simulink model "MoordynSimulinkCoupling_Activefloat"  (R2018b)
settings: Solver=ode45  StartTime=0.0  StopTime=100  RelTol=1e-3
InitFcn:
  | cd 'D:\data\40_mahfouz\Moordyn\MoorDyn v1.01.01'
StartFcn:
  | loadlibrary('MoorDyn','MoorDyn')
StopFcn:
  | calllib('MoorDyn','LinesClose'); % close MoorDyn
  | unloadlibrary MoorDyn; % unload library (never forget to do this!)
CloseFcn:
  | calllib('MoorDyn','LinesClose'); % close MoorDyn
  | unloadlibrary MoorDyn; % unload library (never forget to do this!)
settings Model: Creator=mahfouz  LastModifiedBy=mahfouz
settings DataIOCC: SaveOutput=off  SignalLogging=off  DSMLogging=off  VisualizeSimOutput=off  SaveTime=off
settings OptimizationCC: BlockReduction=off  BooleanDataType=off  ConditionallyExecuteInputs=off  OptimizeBlockIOStorage=off  BufferReuse=off  GlobalBufferReuse=off  ExpressionFolding=off  EnableMemcpy=off  LocalBlockOutputs=off  InitFltsAndDblsToZero=on  EfficientMapNaN2IntZero=off  LifeSpan=inf  OptimizeDataStoreBuffers=off  BusAssignmentInplaceUpdate=off
settings DebuggingCC: SFExecutionAtInitializationDiag=none
settings HardwareCC: TargetBitPerPointer=64  TargetBitPerSizeT=64  TargetBitPerPtrDiffT=64  TargetLongLongMode=on  TargetIntDivRoundTo=Zero  TargetEndianess=LittleEndian  TargetWordSize=64  TargetHWDeviceType=MATLAB Host  ProdEqTarget=off
settings RTWCC: SystemTargetFile=matsim.tlc  PackageName=moordyn  TemplateMakefile=matsim_tmf  Description=Simpack MatSIM Target
settings CodeAppCC: StateflowObjectComments=on
settings STFCustomTargetCC: ModelReferenceCompliant=off  MATLABClassNameForMDSCustomization=Simulink.SoftwareTarget.TargetSpecificTriggerConfigurationBase  GRTInterface=on  SystemTargetFile=matsim.tlc
settings ConfigComp: CovHTMLOptions=-sRT=1 -sVT=0 -aTS=1 -bRG=1 -bTC=1 -hTR=0 -nFC=0 -nFD=1 -scm=1 -bcm=1 -xEv=0 -xEM=0

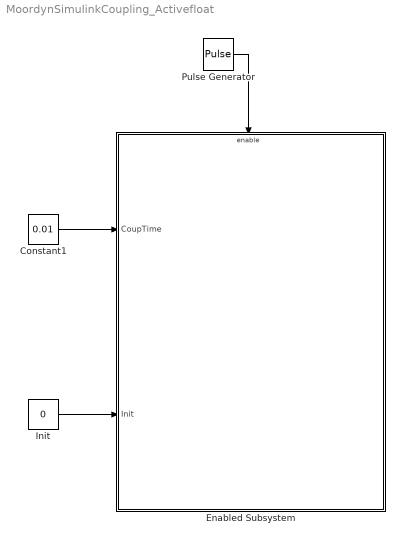
== system MoordynSimulinkCoupling_Activefloat ==
  Constant1 : Constant  Value=0.01
  Enabled Subsystem : Subsystem  TreatAsAtomicUnit=on
  Init : Constant  Value=0
  Pulse Generator : DiscretePulseGenerator  PulseType=Time based  Period=0.01  PulseWidth=70
  wires:
  Constant1/1 -> Enabled Subsystem/1(CoupTime)
  Pulse Generator/1 -> Enabled Subsystem/Enable
  Init/1 -> Enabled Subsystem/2("Init ")

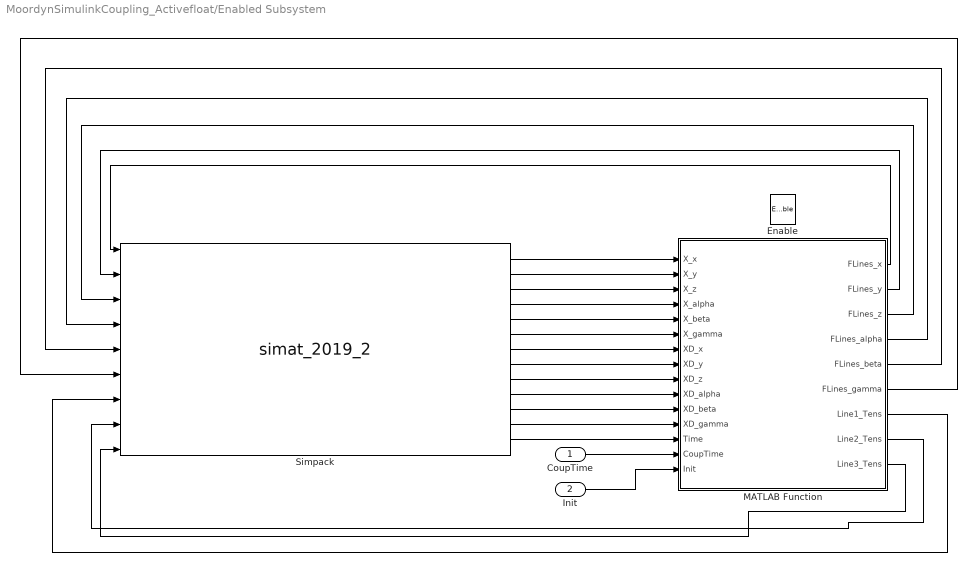
== system MoordynSimulinkCoupling_Activefloat/Enabled Subsystem ==
  CoupTime : Inport
  "Init " : Inport  Port=2
  Enable : EnablePort
  MATLAB Function : MATLAB Function  TreatAsAtomicUnit=on
  Simpack : S-Function  FunctionName=simat_2019_2  Parameters=sample_time server_port server_address auto_start simpack_model initSimpackFirst executionType measType extrapolation_degree singleVectorIO writeSubvarFile writeMFile  SFunctionDeploymentMode=off  EnableBusSupport=off  mask(SIMPACK_SIMAT_2019_2){server_address='localhost', server_port=20104, auto_start=off, simpack_model='m:/my/cosim/model_name.spck', sample_time=0.01, initSimpackFirst=on, executionType=SIMPACK last, measType=on, extrapolation_degree=constant, singleVectorIO=off, resetParameters=off, writeSubvarFile=on, writeMFile=off}
      mask prompts: server_address "Internet address for remote server process"; server_port "TCP-Port of server process"; auto_start "Auto start for SIMPACK Co-Simulation"; simpack_model "SIMPACK model (with full path)"; sample_time "Sampling period"; initSimpackFirst "Init SIMPACK First"; executionType "Execution Type"; measType "Run SIMPACK Measurements"; extrapolation_degree "Extra-/Interpolation"; singleVectorIO "Use one vectorial IO port instead of multiple scalar ones"; resetParameters "Reset parameters to Simpack default values"; writeSubvarFile "Write/Update SIMPACK SubVar file at simulation start (filename: simpack_simat.subvar)"; writeMFile "Write/Update SubVar m-file at SubVar changes (filename: simpack_simat_subvar.m)"
      mask help: Please make sure that either SIMPACK SERVER or SIMPACK COMMAND SERVER is running before any changes are applied.
      mask init:
      | simat_callbacks('MaskInitialization');
      settings: DestroyFcn=simat_callbacks('DestroyFcn');  OpenFcn=simat_callbacks('OpenFcn');
      mask Help:
      | SIMPACK Co-Simulation Interface Version 2019.2 for MATLAB.
      |  This block enables to include SIMPACK MBS model into SIMULINK enviroment.
      | For SIMPACK output file generation, set sampling period to desired nonzero value.
      | S-function simat_2019_2 is required in the Matlab path!
      mask Callback auto_start: simat_callbacks('MaskCallbackString:auto_start');
      mask TypeOptions executionType: parallel | SIMPACK first | SIMPACK last
      mask TypeOptions extrapolation_degree: constant | linear | quadratic | cubic
      mask Callback resetParameters: simat_callbacks('MaskCallbackString:resetParameters');
      mask Display: [dispString, portLabelString] = simat_callbacks('MaskDisplay', '2019.2');disp(dispString);eval(portLabelString);global SPCK_simat_internal_logo_simpack_pic;image(SPCK_simat_internal_logo_simpack_pic, [(1-0.25)/2,1-0.25-0.05,0.25,0.25]);
  wires:
  MATLAB Function/7(Line1_Tens) -> Simpack/7
  MATLAB Function/8(Line2_Tens) -> Simpack/8
  MATLAB Function/9(Line3_Tens) -> Simpack/9
  CoupTime/1 -> MATLAB Function/14(CoupTime)
  Simpack/2 -> MATLAB Function/2(X_y)
  Simpack/1 -> MATLAB Function/1(X_x)
  Simpack/3 -> MATLAB Function/3(X_z)
  Simpack/4 -> MATLAB Function/4(X_alpha)
  Simpack/5 -> MATLAB Function/5(X_beta)
  Simpack/6 -> MATLAB Function/6(X_gamma)
  Simpack/7 -> MATLAB Function/7(XD_x)
  Simpack/8 -> MATLAB Function/8(XD_y)
  Simpack/9 -> MATLAB Function/9(XD_z)
  Simpack/10 -> MATLAB Function/10(XD_alpha)
  Simpack/11 -> MATLAB Function/11(XD_beta)
  Simpack/12 -> MATLAB Function/12(XD_gamma)
  MATLAB Function/2(FLines_y) -> Simpack/2
  MATLAB Function/3(FLines_z) -> Simpack/3
  MATLAB Function/4(FLines_alpha) -> Simpack/4
  MATLAB Function/5(FLines_beta) -> Simpack/5
  MATLAB Function/6(FLines_gamma) -> Simpack/6
  Simpack/13 -> MATLAB Function/13(Time)
  MATLAB Function/1(FLines_x) -> Simpack/1
  "Init "/1 -> MATLAB Function/15(Init)

== matlab function MoordynSimulinkCoupling_Activefloat/Enabled Subsystem/MATLAB Function ==
  data: FLines_x output; FLines_y output; FLines_z output; FLines_alpha output; FLines_beta output; FLines_gamma output; X_x input; X_y input; X_z input; X_alpha input; X_beta input; X_gamma input; XD_x input; XD_y input; XD_z input; XD_alpha input; XD_beta input; XD_gamma input; Time input; CoupTime input; Line1_Tens output; Line2_Tens output; Line3_Tens output; Init input
function [ FLines_x,FLines_y,FLines_z,FLines_alpha,FLines_beta,FLines_gamma,Line1_Tens,Line2_Tens,Line3_Tens ] = MoorDyn(X_x,X_y,X_z,X_alpha,X_beta,X_gamma,XD_x,XD_y,XD_z,XD_alpha,XD_beta,XD_gamma,Time,CoupTime,Init)
coder.extrinsic('MoorDyn_caller')
coder.extrinsic('loadlibrary')
coder.extrinsic('calllib')
coder.extrinsic('cd')
coder.extrinsic('set_param')
coder.extrinsic('find_system')
X = [X_x;X_y;X_z;X_alpha;X_beta;X_gamma];
XD = [XD_x;XD_y;XD_z;XD_alpha;XD_beta;XD_gamma];
if Init == 0 && Time == 0
   calllib('MoorDyn','LinesInit',X,XD);
   set_param('MoordynSimulinkCoupling_Activefloat/Init', 'Value', '1');
elseif Time == 0.01
   set_param('MoordynSimulinkCoupling_Activefloat/Init', 'Value', '0'); 
end

% cd 'D:\data\00_students\4001_Tabea\TabeaRoser\Moordyn\MoorDyn v1.00.03C Source';
 Line1_Tens = 0;
 Line2_Tens = 0;
 Line3_Tens = 0;
 FLines=zeros(1,6);
[ FLines,Line1_Tens,Line2_Tens,Line3_Tens ] = MoorDyn_caller(X,XD,Time,CoupTime);
 FLines_x = -FLines(1);
 FLines_y = -FLines(2);
 FLines_z = -FLines(3);
 FLines_alpha = -FLines(4);
 FLines_beta = -FLines(5);
 FLines_gamma = -FLines(6);
end
